simulink model "arduinotestvol6"  (R2021a)
settings: Solver=FixedStepAuto  StartTime=0.0  StopTime=10.0  RelTol=1e-3
libraries: arduinolib x6
settings Model: SILPILModeSetting=veronly  ExtModeTrigDuration=2  Creator=prime  LastModifiedBy=prime
settings OptimizationCC: EnhancedBackFolding=on  PassReuseOutputArgsAs=Individual arguments  ZeroExternalMemoryAtStartup=off  ZeroInternalMemoryAtStartup=off  MaxStackSize=64  OptimizeBlockOrder=speed  DifferentSizesBufferReuse=on  OptimizationCustomize=off  EfficientTunableParamExpr=on
settings DebuggingCC: ParameterTunabilityLossMsg=error
settings HardwareCC: ProdBitPerPointer=32  ProdBitPerSizeT=32  ProdBitPerPtrDiffT=32  ProdLargestAtomicInteger=Long  ProdLargestAtomicFloat=Double  ProdWordSize=32  ProdHWDeviceType=ARM Compatible->ARM Cortex  UseEmbeddedCoderFeatures=off  UseSimulinkCoderFeatures=off
settings SFSimCC: MATLABDynamicMemAlloc=off
settings RTWCC: SystemTargetFile=ert.tlc  HardwareBoard=Arduino Nano 33 BLE Sense  TemplateMakefile=ert_default_tmf  Toolchain=Arduino ARM MBED  BuildConfiguration=Faster Runs
settings CodeAppCC: ForceParamTrailComments=on  IgnoreCustomStorageClasses=off  OperatorAnnotations=on  SimulinkDataObjDesc=on  SFDataObjDesc=on  InsertBlockDesc=on
settings ERTTargetCC: SupportContinuousTime=on  SupportNonInlinedSFcns=on  SupportVariableSizeSignals=on  ExtModeTransport=3  ExtModeStaticAlloc=on  ExtModeStaticAllocSize=65536  ExtModeMexFile=ext_xcp  ExtModeIntrfLevel=Level2 - Open

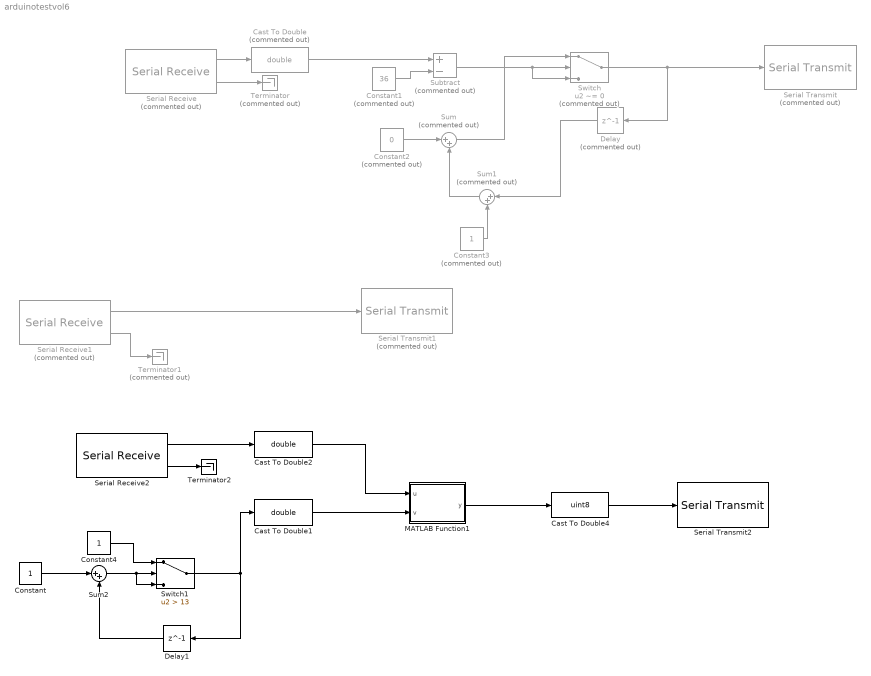
== system arduinotestvol6 ==
  Cast To Double : DataTypeConversion  Commented=on  OutDataTypeStr=double
  Cast To Double1 : DataTypeConversion  OutDataTypeStr=double
  Cast To Double2 : DataTypeConversion  OutDataTypeStr=double
  Cast To Double4 : DataTypeConversion  OutDataTypeStr=uint8
  Constant : Constant
  Constant1 : Constant  Commented=on  Value=36
  Constant2 : Constant  Commented=on  Value=0
  Constant3 : Constant  Commented=on
  Constant4 : Constant
  Delay : Delay  Commented=on  DelayLength=1  InitialCondition=0
  Delay1 : Delay  DelayLength=1  InitialCondition=0
  MATLAB Function1 : MATLAB Function  TreatAsAtomicUnit=on
  Serial Receive : arduinolib/Serial Receive  Commented=on  isARMArch=off  portNumber=1  DataType=uint8  Datalength=1  SampleTime=0.000001  showOutStatus=on  blockPlatform=arduino
      settings: SourceProductBaseCode=ARDUINO
  Serial Receive1 : arduinolib/Serial Receive  Commented=on  isARMArch=off  portNumber=1  DataType=uint8  Datalength=1  SampleTime=0.000001  showOutStatus=on  blockPlatform=arduino
      settings: SourceProductBaseCode=ARDUINO
  Serial Receive2 : arduinolib/Serial Receive  isARMArch=off  portNumber=1  DataType=int8  Datalength=1  SampleTime=0.000001  showOutStatus=on  blockPlatform=arduino
      settings: SourceProductBaseCode=ARDUINO
  Serial Transmit : arduinolib/Serial Transmit  Commented=on  portNumber=0  sendmode=println  sendformat=Decimal  floatprecision=2  blockPlatform=arduino
  Serial Transmit1 : arduinolib/Serial Transmit  Commented=on  portNumber=0  sendmode=println  sendformat=Decimal  floatprecision=2  blockPlatform=arduino
  Serial Transmit2 : arduinolib/Serial Transmit  portNumber=0  sendmode=write  sendformat=Decimal  floatprecision=2  blockPlatform=arduino
  Subtract : Sum  Commented=on  Inputs=+-
  Sum : Sum  Commented=on  Inputs=|++
  Sum1 : Sum  Commented=on  Inputs=|++
  Sum2 : Sum  Inputs=|++
  Switch : Switch  Commented=on  Criteria=u2 ~= 0  Threshold=36
  Switch1 : Switch  Criteria=u2 > Threshold  Threshold=13
  Terminator : Terminator  Commented=on
  Terminator1 : Terminator  Commented=on
  Terminator2 : Terminator
  wires:
  Cast To Double/1 -> Subtract/1
  Constant2/1 -> Sum/1
  Sum/1 -> Switch/1
  Serial Receive/2 -> Terminator/1
  Constant1/1 -> Subtract/2
  Subtract/1 -> Switch/3, Switch/2
  Serial Receive/1 -> Cast To Double/1
  Delay/1 -> Sum1/1
  Constant3/1 -> Sum1/2
  Sum1/1 -> Sum/2
  Switch/1 -> Serial Transmit/1, Delay/1
  Serial Receive1/2 -> Terminator1/1
  MATLAB Function1/1(y) -> Cast To Double4/1
  Serial Receive2/2 -> Terminator2/1
  Cast To Double4/1 -> Serial Transmit2/1
  Constant/1 -> Sum2/1
  Constant4/1 -> Switch1/1
  Switch1/1 -> Delay1/1, Cast To Double1/1
  Sum2/1 -> Switch1/3, Switch1/2
  Delay1/1 -> Sum2/2
  Serial Receive2/1 -> Cast To Double2/1
  Serial Receive1/1 -> Serial Transmit1/1
  Cast To Double1/1 -> MATLAB Function1/2(v)
  Cast To Double2/1 -> MATLAB Function1/1(u)

== matlab function arduinotestvol6/MATLAB Function1 ==
  data: u input; y output; v input
function y  = fcn(u, v)
    if v <= 2
        y = 0;
    else
        y = u;
    end
end
